simulink model "matrix"  (R2018b)
settings: Solver=VariableStepAuto  StartTime=0.0  StopTime=10.0  RelTol=1e-3
model workspace (MAT data in the model file):
  A2 = 4
  B1 = 1
  B2 = 3
  C2 = 2
  D1 = 9
  D2 = 6
  E2 = 7
  F1 = 8
  F2 = 5
settings Model: Creator=Sainquake  LastModifiedBy=Sainquake

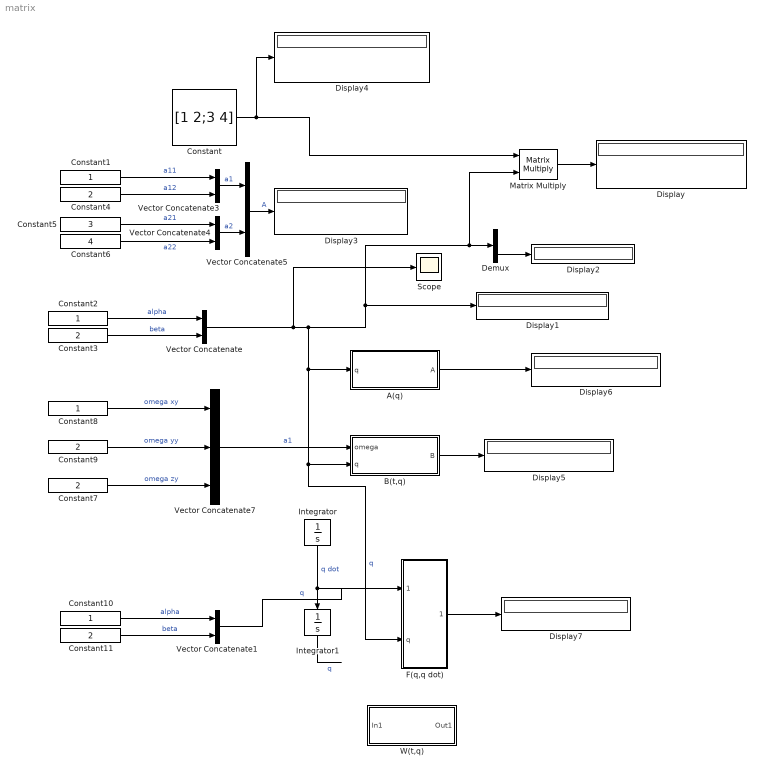
== system matrix ==
  A(q) : Subsystem
  B(t,q) : Subsystem
  Constant : Constant  Value=[1 2;3 4]
  Constant{1..2,8,10} (4 alike) : Constant
  Constant{3..4,7,9,11} (5 alike) : Constant  Value=2
  Constant5 : Constant  Value=3
  Constant6 : Constant  Value=4
  Demux : Demux  Outputs=2
  Display{,1..7} (8 alike) : Display
  F(q,q dot) : Subsystem
  Integrator : Integrator
  Integrator1 : Integrator
  Matrix Multiply : Product  Multiplication=Matrix(*)
  Scope : Scope
  Vector Concatenate{,1,3..5} (5 alike) : Concatenate
  Vector Concatenate7 : Concatenate  NumInputs=3
  W(t,q) : Subsystem
  wires:
  Constant/1 -> Display4/1, Matrix Multiply/1
  Matrix Multiply/1 -> Display/1
  Constant2/1 -> Vector Concatenate/1  "alpha"
  Constant3/1 -> Vector Concatenate/2  "beta"
  Vector Concatenate/1 -> Scope/1, F(q,q dot)/2(q), B(t,q)/2(q), A(q)/1(q), Demux/1, Matrix Multiply/2, Display1/1  "q"
  Demux/2 -> Display2/1
  Constant4/1 -> Vector Concatenate3/2  "a12"
  Constant1/1 -> Vector Concatenate3/1  "a11"
  Constant6/1 -> Vector Concatenate4/2  "a22"
  Constant5/1 -> Vector Concatenate4/1  "a21"
  Vector Concatenate3/1 -> Vector Concatenate5/1  "a1"
  Vector Concatenate4/1 -> Vector Concatenate5/2  "a2"
  Vector Concatenate5/1 -> Display3/1  "A"
  A(q)/1(A) -> Display6/1
  Constant7/1 -> Vector Concatenate7/3  "omega zy"
  Constant8/1 -> Vector Concatenate7/1  "omega xy"
  Constant9/1 -> Vector Concatenate7/2  "omega yy"
  Vector Concatenate7/1 -> B(t,q)/1(omega)  "a1"
  B(t,q)/1(B) -> Display5/1
  Integrator1/1 -> ?  "q"
  Integrator/1 -> Integrator1/1  "q dot"
  ? -> Integrator/1  "q dot dot"
  F(q,q dot)/1(F(q,q dot)) -> Display7/1
  Constant11/1 -> Vector Concatenate1/2  "beta"
  Constant10/1 -> Vector Concatenate1/1  "alpha"
  Vector Concatenate1/1 -> F(q,q dot)/1(q dot)  "q"

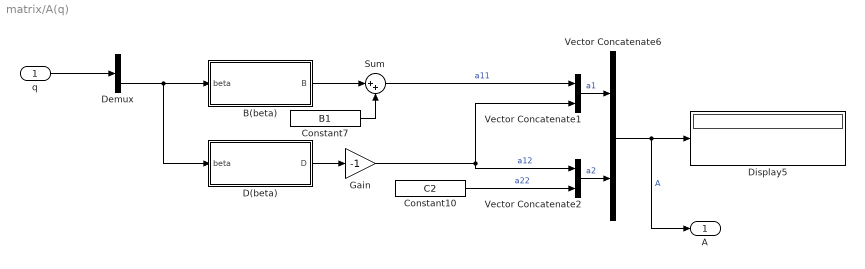
== system matrix/A(q) ==
  q : Inport
  B(beta) : Subsystem
  Constant10 : Constant  Value=C2
  Constant7 : Constant  Value=B1
  D(beta) : Subsystem
  Demux : Demux  Outputs=2
  Display5 : Display
  Gain : Gain  Gain=-1
  Sum : Sum  Inputs=|++
  Vector Concatenate1 : Concatenate
  Vector Concatenate2 : Concatenate
  Vector Concatenate6 : Concatenate
  A : Outport
  wires:
  q/1 -> Demux/1
  Constant7/1 -> Sum/2
  Vector Concatenate2/1 -> Vector Concatenate6/2  "a2"
  Sum/1 -> Vector Concatenate1/1  "a11"
  Constant10/1 -> Vector Concatenate2/2  "a22"
  Vector Concatenate1/1 -> Vector Concatenate6/1  "a1"
  B(beta)/1(B) -> Sum/1
  D(beta)/1(D) -> Gain/1
  Vector Concatenate6/1 -> A/1, Display5/1  "A"
  Gain/1 -> Vector Concatenate1/2, Vector Concatenate2/1  "a12"
  Demux/2 -> D(beta)/1(beta), B(beta)/1(beta)

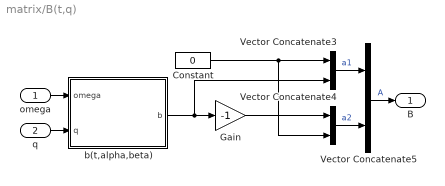
== system matrix/B(t,q) ==
  omega : Inport
  q : Inport  Port=2
  Constant : Constant  Value=0
  Gain : Gain  Gain=-1
  Vector Concatenate3 : Concatenate
  Vector Concatenate4 : Concatenate
  Vector Concatenate5 : Concatenate
  b(t,alpha,beta) : Subsystem
  B : Outport
  wires:
  Vector Concatenate3/1 -> Vector Concatenate5/1  "a1"
  Vector Concatenate5/1 -> B/1  "A"
  Vector Concatenate4/1 -> Vector Concatenate5/2  "a2"
  b(t,alpha,beta)/1(b) -> Vector Concatenate3/2, Gain/1
  Gain/1 -> Vector Concatenate4/1
  Constant/1 -> Vector Concatenate4/2, Vector Concatenate3/1
  omega/1 -> b(t,alpha,beta)/1(omega)
  q/1 -> b(t,alpha,beta)/2(q)

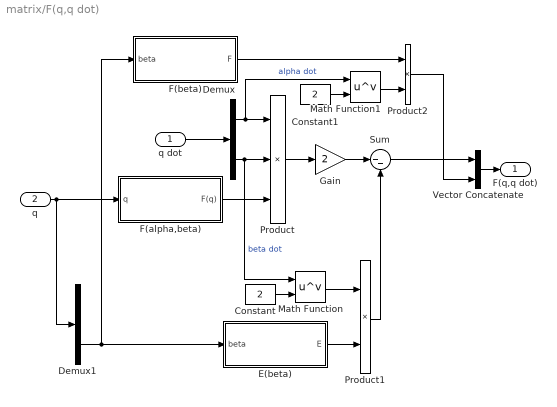
== system matrix/F(q,q dot) ==
  q dot : Inport
  q : Inport  Port=2
  Constant : Constant  Value=2
  Constant1 : Constant  Value=2
  Demux : Demux  Outputs=2
  Demux1 : Demux  Outputs=2
  E(beta) : Subsystem
  F(alpha,beta) : Subsystem
  F(beta) : Subsystem
  Gain : Gain  Gain=2
  Math Function : Math  Operator=pow  SaturateOnIntegerOverflow=on
  Math Function1 : Math  Operator=pow  SaturateOnIntegerOverflow=on
  Product : Product  Inputs=3
  Product1 : Product
  Product2 : Product
  Sum : Sum  Inputs=|--
  Vector Concatenate : Concatenate
  F(q,q dot) : Outport
  wires:
  q dot/1 -> Demux/1
  Product/1 -> Gain/1
  Demux/2 -> Product/2, Math Function/1  "beta dot"
  F(alpha,beta)/1(F(q)) -> Product/3
  q/1 -> F(alpha,beta)/1(q), Demux1/1
  Constant/1 -> Math Function/2
  Math Function/1 -> Product1/1
  E(beta)/1(E) -> Product1/2
  Demux1/2 -> E(beta)/1(beta), F(beta)/1(beta)
  Gain/1 -> Sum/1
  Product1/1 -> Sum/2
  Constant1/1 -> Math Function1/2
  Demux/1 -> Product/1, Math Function1/1  "alpha dot"
  Math Function1/1 -> Product2/2
  F(beta)/1(F) -> Product2/1
  Product2/1 -> Vector Concatenate/2
  Sum/1 -> Vector Concatenate/1
  Vector Concatenate/1 -> F(q,q dot)/1

== system matrix/W(t,q) ==
  In1 : Inport
  Out1 : Outport
  wires:
  In1/1 -> Out1/1

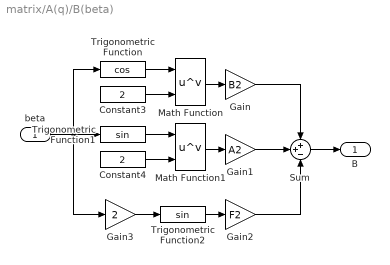
== system matrix/A(q)/B(beta) ==
  beta : Inport
  Constant3 : Constant  Value=2
  Constant4 : Constant  Value=2
  Gain : Gain  Gain=B2
  Gain1 : Gain  Gain=A2
  Gain2 : Gain  Gain=F2
  Gain3 : Gain  Gain=2
  Math Function : Math  Operator=pow  SaturateOnIntegerOverflow=on
  Math Function1 : Math  Operator=pow  SaturateOnIntegerOverflow=on
  Sum : Sum  Inputs=++-
  Trigonometric Function : Trigonometry  Operator=cos
  Trigonometric Function1 : Trigonometry
  Trigonometric Function2 : Trigonometry
  B : Outport
  wires:
  beta/1 -> Gain3/1, Trigonometric Function1/1, Trigonometric Function/1
  Constant3/1 -> Math Function/2
  Trigonometric Function/1 -> Math Function/1
  Math Function/1 -> Gain/1
  Trigonometric Function1/1 -> Math Function1/1
  Math Function1/1 -> Gain1/1
  Constant4/1 -> Math Function1/2
  Trigonometric Function2/1 -> Gain2/1
  Gain3/1 -> Trigonometric Function2/1
  Gain1/1 -> Sum/2
  Gain/1 -> Sum/1
  Gain2/1 -> Sum/3
  Sum/1 -> B/1

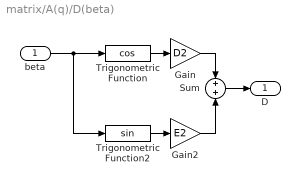
== system matrix/A(q)/D(beta) ==
  beta : Inport
  Gain : Gain  Gain=D2
  Gain2 : Gain  Gain=E2
  Sum : Sum
  Trigonometric Function : Trigonometry  Operator=cos
  Trigonometric Function2 : Trigonometry
  D : Outport
  wires:
  Trigonometric Function/1 -> Gain/1
  Trigonometric Function2/1 -> Gain2/1
  beta/1 -> Trigonometric Function2/1, Trigonometric Function/1
  Gain/1 -> Sum/1
  Sum/1 -> D/1
  Gain2/1 -> Sum/2

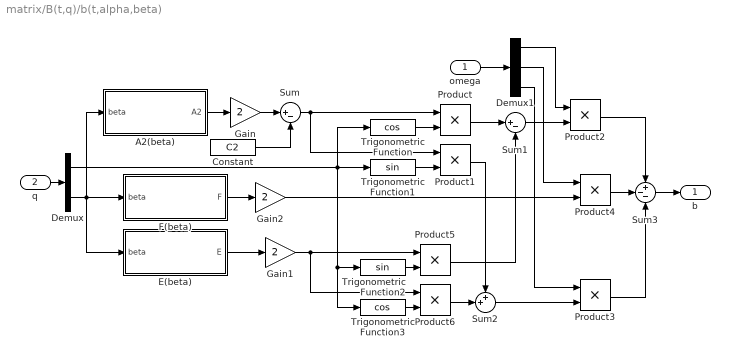
== system matrix/B(t,q)/b(t,alpha,beta) ==
  omega : Inport
  q : Inport  Port=2
  A2(beta) : Subsystem
  Constant : Constant  Value=C2
  Demux : Demux  Outputs=2
  Demux1 : Demux  Outputs=3
  E(beta) : Subsystem
  F(beta) : Subsystem
  Gain : Gain  Gain=2
  Gain1 : Gain  Gain=2
  Gain2 : Gain  Gain=2
  Product{,1..6} (7 alike) : Product
  Sum : Sum  Inputs=|+-
  Sum1 : Sum  Inputs=|+-
  Sum2 : Sum  Inputs=++|
  Sum3 : Sum  Inputs=+--
  Trigonometric Function : Trigonometry  Operator=cos
  Trigonometric Function1 : Trigonometry
  Trigonometric Function2 : Trigonometry
  Trigonometric Function3 : Trigonometry  Operator=cos
  b : Outport
  wires:
  q/1 -> Demux/1
  omega/1 -> Demux1/1
  A2(beta)/1(A2) -> Gain/1
  Constant/1 -> Sum/2
  Gain/1 -> Sum/1
  Sum/1 -> Product1/1, Product/1
  Trigonometric Function/1 -> Product/2
  Demux/1 -> Trigonometric Function3/1, Trigonometric Function2/1, Trigonometric Function1/1, Trigonometric Function/1
  Trigonometric Function1/1 -> Product1/2
  Demux1/1 -> Product2/1
  Trigonometric Function3/1 -> Product6/2
  Trigonometric Function2/1 -> Product5/2
  E(beta)/1(E) -> Gain1/1
  Gain1/1 -> Product6/1, Product5/1
  Demux/2 -> E(beta)/1(beta), A2(beta)/1(beta), F(beta)/1(beta)
  Product/1 -> Sum1/1
  Product5/1 -> Sum1/2
  Product6/1 -> Sum2/2
  Product1/1 -> Sum2/1
  Sum1/1 -> Product2/2
  F(beta)/1(F) -> Gain2/1
  Gain2/1 -> Product4/2
  Demux1/2 -> Product4/1
  Demux1/3 -> Product3/1
  Sum2/1 -> Product3/2
  Product2/1 -> Sum3/1
  Product4/1 -> Sum3/2
  Product3/1 -> Sum3/3
  Sum3/1 -> b/1

== system matrix/F(q,q dot)/E(beta) ==
  beta : Inport
  Gain : Gain  Gain=E2
  Gain2 : Gain  Gain=D2
  Sum : Sum  Inputs=+-
  Trigonometric Function : Trigonometry  Operator=cos
  Trigonometric Function2 : Trigonometry
  E : Outport
  wires:
  Trigonometric Function/1 -> Gain/1
  Trigonometric Function2/1 -> Gain2/1
  beta/1 -> Trigonometric Function2/1, Trigonometric Function/1
  Gain/1 -> Sum/1
  Sum/1 -> E/1
  Gain2/1 -> Sum/2

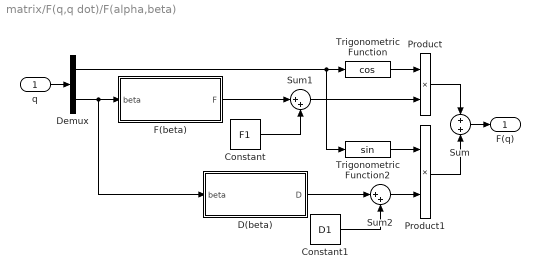
== system matrix/F(q,q dot)/F(alpha,beta) ==
  q : Inport
  Constant : Constant  Value=F1
  Constant1 : Constant  Value=D1
  D(beta) : Subsystem
  Demux : Demux  Outputs=2
  F(beta) : Subsystem
  Product : Product
  Product1 : Product
  Sum : Sum
  Sum1 : Sum  Inputs=|++
  Sum2 : Sum  Inputs=|++
  Trigonometric Function : Trigonometry  Operator=cos
  Trigonometric Function2 : Trigonometry
  F(q) : Outport
  wires:
  Trigonometric Function2/1 -> Product1/1
  Product1/1 -> Sum/2
  Trigonometric Function/1 -> Product/1
  Product/1 -> Sum/1
  Demux/1 -> Trigonometric Function2/1, Trigonometric Function/1
  Sum/1 -> F(q)/1
  F(beta)/1(F) -> Sum1/1
  Constant/1 -> Sum1/2
  Sum1/1 -> Product/2
  Demux/2 -> D(beta)/1(beta), F(beta)/1(beta)
  D(beta)/1(D) -> Sum2/1
  Constant1/1 -> Sum2/2
  Sum2/1 -> Product1/2
  q/1 -> Demux/1

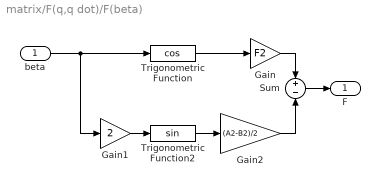
== system matrix/F(q,q dot)/F(beta) ==
  beta : Inport
  Gain : Gain  Gain=F2
  Gain1 : Gain  Gain=2
  Gain2 : Gain  Gain=(A2-B2)/2
  Sum : Sum  Inputs=+-
  Trigonometric Function : Trigonometry  Operator=cos
  Trigonometric Function2 : Trigonometry
  F : Outport
  wires:
  Trigonometric Function/1 -> Gain/1
  Trigonometric Function2/1 -> Gain2/1
  beta/1 -> Trigonometric Function/1, Gain1/1
  Gain/1 -> Sum/1
  Sum/1 -> F/1
  Gain2/1 -> Sum/2
  Gain1/1 -> Trigonometric Function2/1

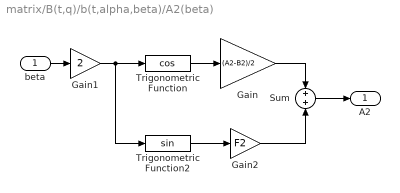
== system matrix/B(t,q)/b(t,alpha,beta)/A2(beta) ==
  beta : Inport
  Gain : Gain  Gain=(A2-B2)/2
  Gain1 : Gain  Gain=2
  Gain2 : Gain  Gain=F2
  Sum : Sum
  Trigonometric Function : Trigonometry  Operator=cos
  Trigonometric Function2 : Trigonometry
  A2 : Outport
  wires:
  Trigonometric Function/1 -> Gain/1
  Trigonometric Function2/1 -> Gain2/1
  beta/1 -> Gain1/1
  Gain/1 -> Sum/1
  Sum/1 -> A2/1
  Gain2/1 -> Sum/2
  Gain1/1 -> Trigonometric Function2/1, Trigonometric Function/1

== system matrix/B(t,q)/b(t,alpha,beta)/E(beta) ==
  beta : Inport
  Gain : Gain  Gain=E2
  Gain2 : Gain  Gain=D2
  Sum : Sum  Inputs=+-
  Trigonometric Function : Trigonometry  Operator=cos
  Trigonometric Function2 : Trigonometry
  E : Outport
  wires:
  Trigonometric Function/1 -> Gain/1
  Trigonometric Function2/1 -> Gain2/1
  beta/1 -> Trigonometric Function2/1, Trigonometric Function/1
  Gain/1 -> Sum/1
  Sum/1 -> E/1
  Gain2/1 -> Sum/2

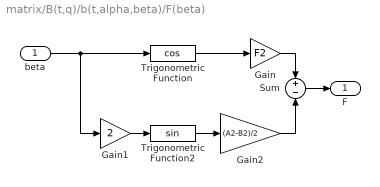
== system matrix/B(t,q)/b(t,alpha,beta)/F(beta) ==
  beta : Inport
  Gain : Gain  Gain=F2
  Gain1 : Gain  Gain=2
  Gain2 : Gain  Gain=(A2-B2)/2
  Sum : Sum  Inputs=+-
  Trigonometric Function : Trigonometry  Operator=cos
  Trigonometric Function2 : Trigonometry
  F : Outport
  wires:
  Trigonometric Function/1 -> Gain/1
  Trigonometric Function2/1 -> Gain2/1
  beta/1 -> Trigonometric Function/1, Gain1/1
  Gain/1 -> Sum/1
  Sum/1 -> F/1
  Gain2/1 -> Sum/2
  Gain1/1 -> Trigonometric Function2/1

== system matrix/F(q,q dot)/F(alpha,beta)/D(beta) ==
  beta : Inport
  Gain : Gain  Gain=D2
  Gain2 : Gain  Gain=E2
  Sum : Sum
  Trigonometric Function : Trigonometry  Operator=cos
  Trigonometric Function2 : Trigonometry
  D : Outport
  wires:
  Trigonometric Function/1 -> Gain/1
  Trigonometric Function2/1 -> Gain2/1
  beta/1 -> Trigonometric Function2/1, Trigonometric Function/1
  Gain/1 -> Sum/1
  Sum/1 -> D/1
  Gain2/1 -> Sum/2

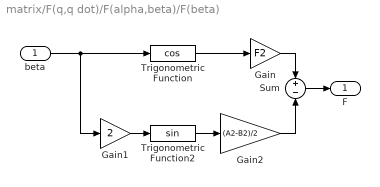
== system matrix/F(q,q dot)/F(alpha,beta)/F(beta) ==
  beta : Inport
  Gain : Gain  Gain=F2
  Gain1 : Gain  Gain=2
  Gain2 : Gain  Gain=(A2-B2)/2
  Sum : Sum  Inputs=+-
  Trigonometric Function : Trigonometry  Operator=cos
  Trigonometric Function2 : Trigonometry
  F : Outport
  wires:
  Trigonometric Function/1 -> Gain/1
  Trigonometric Function2/1 -> Gain2/1
  beta/1 -> Trigonometric Function/1, Gain1/1
  Gain/1 -> Sum/1
  Sum/1 -> F/1
  Gain2/1 -> Sum/2
  Gain1/1 -> Trigonometric Function2/1
